simulink model "licimox"  (R2014a)
settings: Solver=ode45  StartTime=0.0  StopTime=10.0  RelTol=1e-3
settings Model: Creator=ztg  LastModifiedBy=ztg

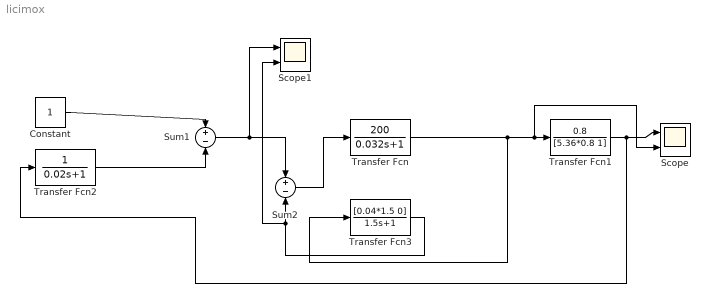
== system licimox ==
  Constant : Constant
  Scope : Scope  NumInputPorts=2
      settings: YMin=0~0  YMax=1.5~1.5
  Scope1 : Scope  NumInputPorts=2
      settings: YMin=0~0  YMax=1.5~1.5
  Sum1 : Sum  Inputs=+-
  Sum2 : Sum  Inputs=+-
  Transfer Fcn : TransferFcn  Numerator=[200]  Denominator=[0.032 1]
  Transfer Fcn1 : TransferFcn  Numerator=[0.8]  Denominator=[5.36*0.8 1]
  Transfer Fcn2 : TransferFcn  Denominator=[0.02 1]
  Transfer Fcn3 : TransferFcn  Numerator=[0.04*1.5 0]  Denominator=[1.5 1]
  wires:
  Constant/1 -> Sum1/1
  Sum1/1 -> Scope1/1, Sum2/1
  Transfer Fcn2/1 -> Sum1/2
  Transfer Fcn1/1 -> Transfer Fcn2/1, Scope/1
  Transfer Fcn/1 -> Transfer Fcn3/1, Scope/2, Transfer Fcn1/1
  Transfer Fcn3/1 -> Scope1/2, Sum2/2
  Sum2/1 -> Transfer Fcn/1
